simulink model "first2"  (R2014b)
settings: Solver=ode45  StartTime=0.0  StopTime=30  MaxStep=0.001  MinStep=0.0001  RelTol=1e-3
libraries: simulink x2
settings Model: Creator=Игорь  LastModifiedBy=Игорь

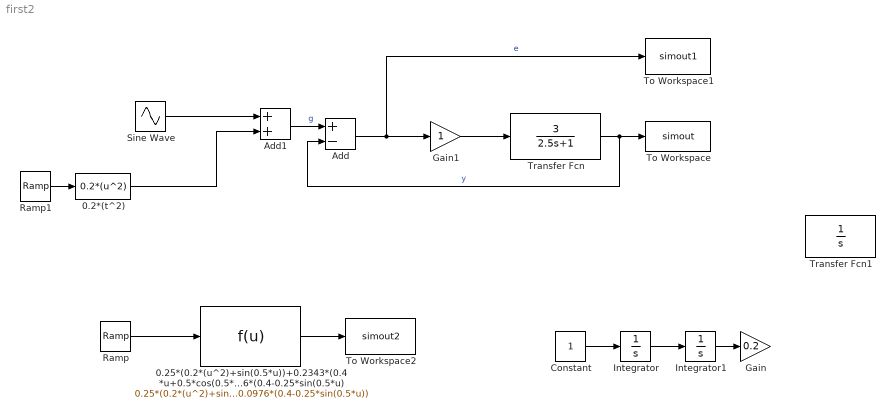
== system first2 ==
  0.2*(t^2) : Fcn  Expr=0.2*(u^2)
  0.25*(0.2*(u^2)+sin(0.5*u))+0.2343*(0.4*u+0.5*cos(0.5*u))+0.0976*(0.4-0.25*sin(0.5*u) : Fcn  Expr=0.25*(0.2*(u^2)+sin(0.5*u))+0.2343*(0.4*u+0.5*cos(0.5*u))+0.0976*(0.4-0.25*sin(0.5*u))
  Add : Sum  Inputs=+-
  Add1 : Sum
  Constant : Constant
  Gain : Gain  Gain=0.2
  Gain1 : Gain
  Integrator : Integrator
  Integrator1 : Integrator
  Ramp : simulink/Sources/Ramp  slope=1  start=0  X0=0
  Ramp1 : simulink/Sources/Ramp  slope=1  start=0  X0=0
  Sine Wave : Sin  Frequency=0.5  SampleTime=0
  To Workspace : ToWorkspace  VariableName=simout  SaveFormat=Timeseries  SampleTime=-1
  To Workspace1 : ToWorkspace  VariableName=simout1  SaveFormat=Timeseries  SampleTime=-1
  To Workspace2 : ToWorkspace  VariableName=simout2  SaveFormat=Timeseries  SampleTime=-1
  Transfer Fcn : TransferFcn  Numerator=[3]  Denominator=[2.5 1]
  Transfer Fcn1 : TransferFcn  Denominator=[1 0]
  wires:
  Transfer Fcn/1 -> Add/2, To Workspace/1  "y"
  Add/1 -> Gain1/1, To Workspace1/1  "e"
  Integrator/1 -> Integrator1/1
  Constant/1 -> Integrator/1
  Integrator1/1 -> Gain/1
  Gain1/1 -> Transfer Fcn/1
  Sine Wave/1 -> Add1/1
  Add1/1 -> Add/1  "g"
  0.25*(0.2*(u^2)+sin(0.5*u))+0.2343*(0.4*u+0.5*cos(0.5*u))+0.0976*(0.4-0.25*sin(0.5*u)/1 -> To Workspace2/1
  Ramp/1 -> 0.25*(0.2*(u^2)+sin(0.5*u))+0.2343*(0.4*u+0.5*cos(0.5*u))+0.0976*(0.4-0.25*sin(0.5*u)/1
  Ramp1/1 -> 0.2*(t^2)/1
  0.2*(t^2)/1 -> Add1/2
